simulink model "P3GPID"  (Simulink 8.5)
settings: Solver=ode5  StartTime=0.0  StopTime=10.0  FixedStep=0.01  RelTol=1e-3
values from neighbouring files (symbols this model uses):
  Kd = chro(3)    [GA_fitfun_P3PID.m]    (also in P3PID.m = minimum_Kp_Ki_Kd(3); P3PID_rp.m = minimum_Kp_Ki_Kd(3))
  Ki = chro(2)    [GA_fitfun_P3PID.m]    (also in P3PID.m = minimum_Kp_Ki_Kd(2); P3PID_rp.m = minimum_Kp_Ki_Kd(2))
  Kp = chro(1)    [GA_fitfun_P3PID.m]    (also in P3PID.m = minimum_Kp_Ki_Kd(1); P3PID_rp.m = minimum_Kp_Ki_Kd(1))
settings Model: Creator=dsp520  LastModifiedBy=dsp520
settings DataIOCC: SignalLoggingSaveFormat=Dataset
settings OptimizationCC: ExpressionDepthLimit=128
settings DebuggingCC: UnderspecifiedInitializationDetection=Simplified  MergeDetectMultiDrivingBlocksExec=error  FcnCallInpInsideContextMsg=EnableAllAsError  StateNameClashWarn=none
settings GRTTargetCC: CombineOutputUpdateFcns=on  GRTInterface=off

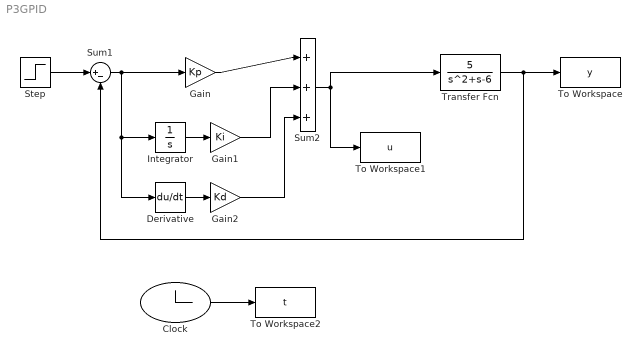
== system P3GPID ==
  Clock : Clock
  Derivative : Derivative
  Gain : Gain  Gain=Kp
  Gain1 : Gain  Gain=Ki
  Gain2 : Gain  Gain=Kd
  Integrator : Integrator
  Step : Step  Time=0  SampleTime=0
  Sum1 : Sum  Inputs=|+-
  Sum2 : Sum  Inputs=|+++
  To Workspace : ToWorkspace  VariableName=y  SampleTime=-1
  To Workspace1 : ToWorkspace  VariableName=u  SampleTime=-1
  To Workspace2 : ToWorkspace  VariableName=t  SampleTime=-1
  Transfer Fcn : TransferFcn  Numerator=[5]  Denominator=[1 1 -6]
  wires:
  Step/1 -> Sum1/1
  Integrator/1 -> Gain1/1
  Derivative/1 -> Gain2/1
  Sum1/1 -> Derivative/1, Integrator/1, Gain/1
  Gain/1 -> Sum2/1
  Gain1/1 -> Sum2/2
  Gain2/1 -> Sum2/3
  Sum2/1 -> Transfer Fcn/1, To Workspace1/1
  Clock/1 -> To Workspace2/1
  Transfer Fcn/1 -> Sum1/2, To Workspace/1
